simulink model "log_data"  (R2016b)
settings: Solver=FixedStepDiscrete  StartTime=0.0  StopTime=10.0  RelTol=1e-3
libraries: pixhawk_slib_sensors_actuators x3, pixhawk_slib_misc_utils x1
settings Model: Creator=Mr Wang  LastModifiedBy=Mr Wang
settings OptimizationCC: DefaultParameterBehavior=Inlined  MaxStackSize=64
settings DebuggingCC: ParameterTunabilityLossMsg=error
settings HardwareCC: ProdBitPerPointer=32  ProdBitPerSizeT=32  ProdBitPerPtrDiffT=32  ProdLargestAtomicInteger=Long  ProdLargestAtomicFloat=Double  ProdWordSize=32  ProdHWDeviceType=ARM Compatible->ARM Cortex
settings RTWCC: SystemTargetFile=ert.tlc  HardwareBoard=Pixhawk PX4  TLCOptions="-aInlineSetEventsForThisBaseRateFcn=TLC_FALSE -aSuppressMultiTaskScheduler=TLC_FALSE  -aRateBasedStepFcn=0"  TemplateMakefile=ert_default_tmf  Description=Embedded Coder  GenerateReport=on  Toolchain=Pixhawk Toolchain  IncludeHyperlinkInReport=on  LaunchReport=on  GenerateTraceInfo=on  GenerateTraceReport=on  GenerateTraceReportSl=on  GenerateTraceReportSf=on  GenerateTraceReportEml=on
settings CodeAppCC: ForceParamTrailComments=on  IgnoreCustomStorageClasses=off  OperatorAnnotations=on  SimulinkDataObjDesc=on  SFDataObjDesc=on  MATLABFcnDesc=on  InsertBlockDesc=on  MATLABSourceComments=on
settings ERTTargetCC: ERTCustomFileTemplate=PX4_codertarget_file_process.tlc

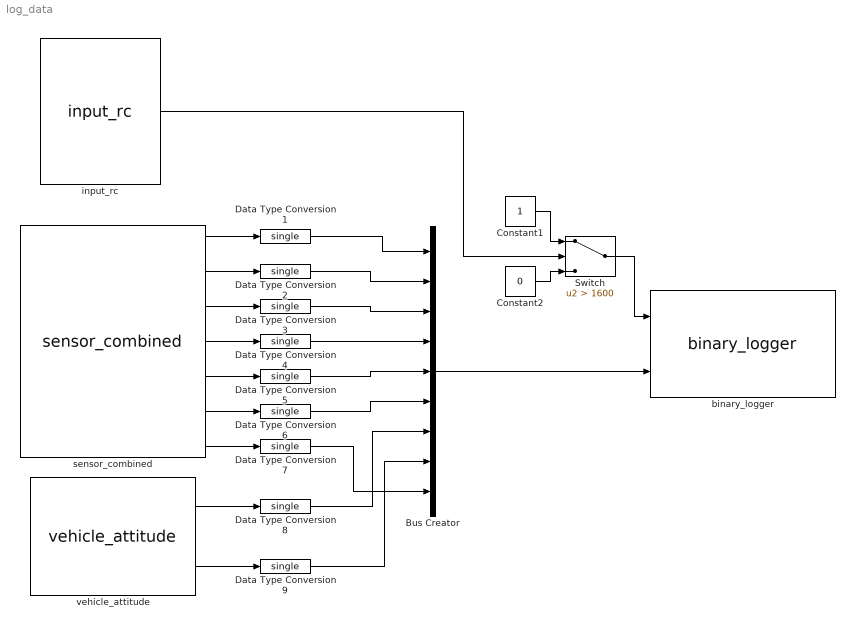
== system log_data ==
  Bus Creator : BusCreator  Inputs=9
  Constant1 : Constant  OutDataTypeStr=boolean  SampleTime=1
  Constant2 : Constant  Value=0  OutDataTypeStr=boolean  SampleTime=1
  Data Type Conversion{1..9} (9 alike) : DataTypeConversion  OutDataTypeStr=single
  Switch : Switch  Criteria=u2 > Threshold  Threshold=1600
  binary_logger : pixhawk_slib_misc_utils/binary_logger  logfile=/fs/microsd/log/e4  cacheflag=off  numRecs=60000
  input_rc : pixhawk_slib_sensors_actuators/input_rc  sampletime=1/250  channel1=off  channel2=off  channel3=off  channel4=off  channel5=on  channel6=off  channel7=off  channel8=off  ch_count=off  rssi=off  rc_failsafe=off  rc_lost=off  rc_inputsource=off
  sensor_combined : pixhawk_slib_sensors_actuators/sensor_combined  sampletime=1/250  show_mag=off  show_acc=on  show_gyro=on  show_baro=off  show_ts=on
  vehicle_attitude : pixhawk_slib_sensors_actuators/vehicle_attitude  sampletime=1/250  show_r=on  show_p=on  show_y=off  show_q=off
  wires:
  input_rc/1 -> Switch/2
  sensor_combined/4 -> Data Type Conversion4/1
  sensor_combined/6 -> Data Type Conversion6/1
  vehicle_attitude/1 -> Data Type Conversion8/1
  vehicle_attitude/2 -> Data Type Conversion9/1
  sensor_combined/5 -> Data Type Conversion5/1
  Data Type Conversion1/1 -> Bus Creator/1
  Data Type Conversion2/1 -> Bus Creator/2
  Data Type Conversion3/1 -> Bus Creator/3
  Data Type Conversion4/1 -> Bus Creator/4
  Data Type Conversion5/1 -> Bus Creator/5
  Data Type Conversion6/1 -> Bus Creator/6
  Data Type Conversion8/1 -> Bus Creator/7
  Data Type Conversion9/1 -> Bus Creator/8
  Data Type Conversion7/1 -> Bus Creator/9
  sensor_combined/1 -> Data Type Conversion1/1
  sensor_combined/2 -> Data Type Conversion2/1
  sensor_combined/3 -> Data Type Conversion3/1
  sensor_combined/7 -> Data Type Conversion7/1
  Bus Creator/1 -> binary_logger/2
  Constant1/1 -> Switch/1
  Switch/1 -> binary_logger/1
  Constant2/1 -> Switch/3
